simulink model "myRIo_block"  (R2023b)
settings: Solver=VariableStepAuto  StartTime=0.0  StopTime=0.5  RelTol=1e-3
libraries: simulink x6
settings Model: Creator=joeas  LastModifiedBy=joeas

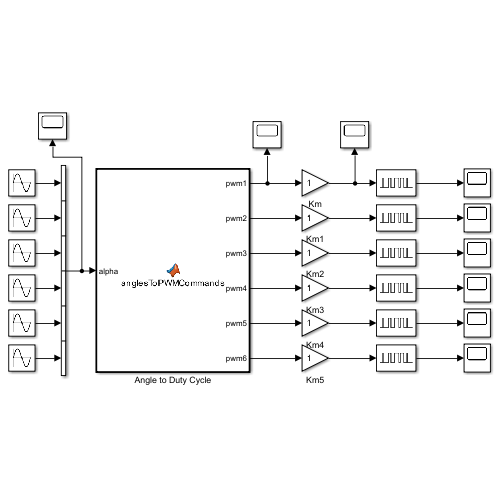
[thumbnail: Simulink's stored preview of the top-level diagram]
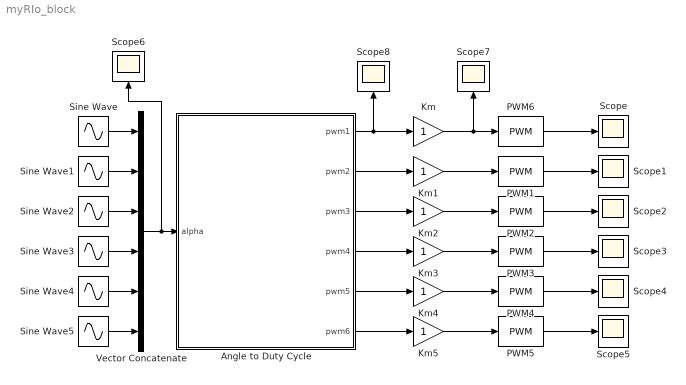
== system myRIo_block ==
  Angle to Duty Cycle : MATLAB Function  TreatAsAtomicUnit=on
  Km{,1..5} (6 alike) : Gain
  PWM{1..6} (6 alike) : simulink/Discontinuities/PWM  DisableCoverage=on  Period=1  InitialDelay=0  DisallowZeroDutyCycle=off  RunAtFixedTimeIntervals=off  SampleTime=0.1
  Scope{,1..8} (9 alike) : Scope
  Sine Wave : Sin  Amplitude=3  SampleTime=0
  Sine Wave{1..5} (5 alike) : Sin  SampleTime=0
  Vector Concatenate : Concatenate  NumInputs=6
  wires:
  Angle to Duty Cycle/1(pwm1) -> Km/1, Scope8/1
  Km/1 -> PWM6/1, Scope7/1
  Vector Concatenate/1 -> Scope6/1, Angle to Duty Cycle/1(alpha)
  Km1/1 -> PWM1/1
  Angle to Duty Cycle/2(pwm2) -> Km1/1
  PWM1/1 -> Scope1/1
  Km2/1 -> PWM2/1
  Angle to Duty Cycle/3(pwm3) -> Km2/1
  PWM2/1 -> Scope2/1
  Km3/1 -> PWM3/1
  Angle to Duty Cycle/4(pwm4) -> Km3/1
  PWM3/1 -> Scope3/1
  Km4/1 -> PWM4/1
  Angle to Duty Cycle/5(pwm5) -> Km4/1
  PWM4/1 -> Scope4/1
  Km5/1 -> PWM5/1
  Angle to Duty Cycle/6(pwm6) -> Km5/1
  PWM5/1 -> Scope5/1
  Sine Wave/1 -> Vector Concatenate/1
  Sine Wave4/1 -> Vector Concatenate/5
  Sine Wave1/1 -> Vector Concatenate/2
  Sine Wave2/1 -> Vector Concatenate/3
  Sine Wave3/1 -> Vector Concatenate/4
  Sine Wave5/1 -> Vector Concatenate/6
  PWM6/1 -> Scope/1

== matlab function myRIo_block/Angle to Duty Cycle ==
  data: alpha input; pwm1 output; pwm2 output; pwm3 output; pwm4 output; pwm5 output; pwm6 output
function [pwm1, pwm2, pwm3, pwm4, pwm5, pwm6]  = anglesToPWMCommands(alpha)
% Function to map an array of servo angles to PWM commands
% angles: A vector containing the desired angles for each servo
% pwmCommands: A vector containing the PWM commands for each servo

% Initialize output vector
pwmCommands = zeros(1, length(alpha));

% Servo specs
minAngle = 0;   % degrees
maxAngle = 180; % degrees
minPulse = 1;   % Pulse width in ms
maxPulse = 2;   % Pulse width in ms

% Calculate PWM commands
for i = 1:length(alpha)
    angle = alpha(i);
    pulseWidth = (angle - minAngle) * (maxPulse - minPulse) / (maxAngle - minAngle) + minPulse;
    pwmCommands(i) = (pulseWidth / 20) * 100; % Convert pulse width to duty cycle percentage
end

pwm1 = pwmCommands(1);
pwm2 = pwmCommands(2);
pwm3 = pwmCommands(3);
pwm4 = pwmCommands(4);
pwm5 = pwmCommands(5);
pwm6 = pwmCommands(6);

end
